simulink model "MGTestSystem_4bus"  (R2021b)
settings: Solver=VariableStepAuto  StartTime=0.0  StopTime=4  RelTol=1e-3
PreLoadFcn:
  | addpath Icons
  | addpath Util
InitFcn:
  | clc
  | %clear all
  | 
  | nDER = 4;
  | xssum = zeros(nDER*2,1);
  | save XSSUM xssum
  | 
  | Ts_Control=1e-4;       % local control time step
  | Ts_Simulation=5e-5;   %simulation time step
  | Ts_Power=5e-5;   % measurement time step
  | Tdisc=0.8;     % time setting for disconnecting from the main grid
  | 
  | Iref = 0.3;  % in p.u.
  | Iqref = 0;  % in p.u.
  | 
  | Ts_secondary =3e-2;   %  secondary control time step
  | %Ts_PMU = 1/60;
  | 
  | ft2km=3.0480e-04;
  | 
  | KPdroop=3.4e-4;
  | KQdroop=1e-3/1;
  | KPdroop2=4.5e-4;
  | KQdroop2=1.5e-3/1;
  | 
  | %KWinvdroop = 20.0;
  | %KVinvdroop = 16.7;
  | %KWinvdroop = 0.05;
  | %KVinvdroop = 0.08;
  | 
  | KWinvdroop = 1/(2*pi*KPdroop);
  | KVinvdroop = 1/(2*pi*KQdroop)
  | KWinvdroop2 = 1/(2*pi*KPdroop2);
  | KVinvdroop2 = 1/(2*pi*KQdroop2)
  | %KVinvdroop = 1/(KQdroop);
  | %KVinvdroop2 = 1/(KQdroop2);
  | %KWinvdroop = 1/(KPdroop);
  | %KWinvdroop2 = 1/(KPdroop2);
  | 
  | droopv1=1/KVinvdroop
  | droopv2=1/KVinvdroop2
  | 
  | 
  | 
  | 
  | wfilter = 35;
  | Rv=0.0;
  | Lv=0e-3;
  | 
  | div=1;
  | 
  | 
  | Kpac=0.1/1;
  | Kiac=420/1;
  | Kpaci=15/div;
  | Kiaci=2e3/div;
  | Kpac2=0.05/1;
  | Kiac2=390/1;
  | Kpaci2=15/div;
  | Kiaci2=1.6e3/div;
  | ... (+47 lines)
undefined symbols (not defined in the file or in its folder): D1, Delta, Ion, Lithium
libraries: spsStairGeneratorLib x24, spsThreePhaseSeriesRLCBranchLib x24, powerlib_extras x23, spsSeriesRLCBranchLib x20, spsThreePhaseVIMeasurementLib x18, slpidlib x18, spsThreePhaseBreakerLib x15, spsRMSLib x10, spsThreePhaseSeriesRLCLoadLib x8, spsVoltageMeasurementLib x8, spsPMUPLLBasedPositiveSequenceLib x6, spsPowerLib x5
(part 2 of 7)

== system MGTestSystem_4bus/DER 1 ==
  Battery : spsBatteryLib/Battery  Commented=on  BatType=Lithium-Ion  ShowTempParam=off  ThermalPreset=no  ShowAgeParam=off  NomV=960  NomQ=10  SOC=75  Batt_Tr=30  PresetModel=on  MaxQ=10  MinV=720  FullV=1117.4277  Dis_rate=4.3478  R=0.96  Normal_OP=9.0435  expZone="[1037.1704     0.49130435]"  current=[6.5 13 32.5]  Units=Time  Tci=20  NomT=20  T2=-30  MaxQ2=4.8  FullV2=7.1  Normal_OP2=5.655  expZone2="[6.58           1]"  Rca=0.6  ti=2000  Dp=0  Neq0=0  Tsim=1e6  Ta1=25  Qeol=5.4*0.9  Reol=0.013333*1.2  Char_age=[2.3478, 3]  Dis_age=[2.3478, 10]  N1=1500  N2=10500  N3=1000  N4=1400  Ta2=45  N5=950
  C1 : spsSeriesRLCBranchLib/Series RLC Branch  LConnTagsString=__new0  RConnTagsString=__new0  BranchType=C  Resistance=1.0  Inductance=1.0  SetiL0=off  InitialCurrent=0  Capacitance=50e-3  Setx0=off  InitialVoltage=960  Measurements=None
  C2 : spsSeriesRLCBranchLib/Series RLC Branch  LConnTagsString=__new0  RConnTagsString=__new0  BranchType=R  Resistance=1e-9  Inductance=1.0  SetiL0=off  InitialCurrent=0  Capacitance=200e-3  Setx0=on  InitialVoltage=500  Measurements=None
  DC Voltage Source : spsDCVoltageSourceLib/DC Voltage Source  Amplitude=VDC  Measurements=None
  DC/DC 1 : Subsystem  Commented=on
  Demux : Demux  Commented=on  Outputs=3
  Irradiance (W/m2) 1 : spsStairGeneratorLib/Stair Generator  Commented=on  t=[0, 10.5, 12.3]  e=[1,0.05, 1.0]*1000  Ts=Ts_Power
  L : spsThreePhaseSeriesRLCBranchLib/Three-Phase Series RLC Branch  LConnTagsString=A|B|C  RConnTagsString=A|B|C  BranchType=RL  Resistance=0.1  Inductance=1.35e-3  Capacitance=inf  Measurements=None
  L1 : spsThreePhaseSeriesRLCBranchLib/Three-Phase Series RLC Branch  LConnTagsString=A|B|C  RConnTagsString=A|B|C  BranchType=RC  Resistance=1  Inductance=3.9e-3  Capacitance=50e-6  Measurements=None
  L3 : spsThreePhaseSeriesRLCBranchLib/Three-Phase Series RLC Branch  Commented=on  LConnTagsString=A|B|C  RConnTagsString=A|B|C  BranchType=RL  Resistance=0*0.03  Inductance=0*0.35e-3  Capacitance=1e-9  Measurements=None
  Local bus : spsThreePhaseVIMeasurementLib/Three-Phase V-I Measurement  VoltageMeasurement=phase-to-ground  SetLabelV=off  LabelV=Vgrid  Vpu=off  VpuLL=off  CurrentMeasurement=yes  SetLabelI=off  LabelI=Igrid  Ipu=off  Pbase=100e6  Vbase=500e3  OutputType=Magnitude  PhasorSimulation=off  PSBequivalent=0
  PV Array 1 : spsPVArrayLib/PV Array  Commented=on  Npar=32  Nser=3  PlotType=array @ 1000 W/m2 & specified temperatures  S_vec="[ 1000  500  100 ]"  Temp_C_vec="[ 45 25  ]"  ModuleName=SunPower SPR-315E-WHT-D  PlotWhenSelected=off  Pm=315.072  Ncell=96  Voc=64.6  Isc=6.14  Vm=54.7  Im=5.76  beta_Voc_pc=-0.2727  alpha_Isc_pc=0.061743  beta_Voc=-0.17616  alpha_Isc=0.003791  IL=6.1461  I0=6.5067e-12  nI=0.95071  Rsh=430.0666  Rs=0.43041  RobustModel=off  RobustCellTemperature=313.3991  BAL=off  Tc=1e-6  Tfilter=5e-5
  Rate Limiter2 : RateLimiter  Commented=on  RisingSlewLimit=8000  FallingSlewLimit=-8000  SampleTimeMode=inherited  InitialCondition=1000
  Scope : Scope
  Scope1 : Scope
  Scope2 : Scope  Commented=on  NumInputPorts=3
  VSC (Average Model) : spsUniversalBridgeLib/Universal Bridge  Arms=3  SnubberResistance=1e5  SnubberCapacitance=inf  Device=Average-model based VSC  Ron=1e-3  Lon=0  ForwardVoltages="[  0  0  ]"  ForwardVoltage=0  GTOparameters=[ 10e-6 , 20e-6 ]  IGBTparameters=[ 1e-6 , 2e-6 ]  Measurements=None  Measurements_2=None  converterType=Rectifier
  VSC Control : Subsystem  mask(VSC Main Controller){nom=[ Pvscr 60 ], Vnom=[480 480], Vnom_dc=VDC, RLxfo=[0*0.03*Pvscr/(480^2)  0*0.35e-3*Pvscr/(480^2)*2*pi*60], RLchoke=[0.08  1.35e-3 ], K_VDCreg=[7  800], K_Ireg=[Kpaci Kiaci], Ts=Ts_Control}
      mask prompts: nom "Nominal power and frequency [ Pnom(VA)  Fnom(Hz) ]:"; Vnom "Nominal primary and secondary voltages (Vrms LL) [ Vnom_prim   Vnom_sec ]:"; Vnom_dc "Nominal DC bus voltage (V):"; RLxfo "Total transformer leakage impedance (pu/Pnom) [ Rxfo  Lxf ]"; RLchoke "Choke impedance [ R(ohm) L(H) ]"; K_VDCreg "VDC regultator gains [ Kp  Ki ]:"; K_Ireg "Current regulator gains [ Kp  Ki ]:"; Ts "Sample time"
      mask init:
      | Pnom=nom(1);
      | Fnom=nom(2);
      | Vnom_prim=Vnom(1);
      | Vnom_sec=Vnom(2);
      | Zbase=Vnom_sec^2/Pnom;
      | Rtot_pu=RLxfo(1) + RLchoke(1)/Zbase;
      | Ltot_pu=RLxfo(2) + RLchoke(2)/(Zbase/(2*pi*Fnom));
      | Kp_VDCreg=K_VDCreg(1);
      | Ki_VDCreg=K_VDCreg(2);
      | Kp_Ireg=K_Ireg(1);
      | Ki_Ireg=K_Ireg(2);
      | Vdc_ref=Vnom_dc;
  "Vdc " : spsVoltageMeasurementLib/Voltage Measurement  Tag=PoWeRsYsTeMmEaSuReMeNt  PhasorSimulation=off  OutputType=Magnitude  PSBequivalent=0
  Conn1 : PMIOPort  Side=Left
  Conn2 : PMIOPort  Port=2  Side=Left
  Conn3 : PMIOPort  Port=3  Side=Left
  wires:
  "Vdc "/1 -> Scope/1, VSC Control/3(Vdc)
  VSC Control/1(Uref) -> Scope1/1, VSC (Average Model)/1
  Local bus/1 -> VSC Control/1(V)
  Local bus/2 -> VSC Control/2(I)
  Irradiance (W/m2) 1/1 -> Rate Limiter2/1
  Rate Limiter2/1 -> PV Array 1/1
  PV Array 1/1 -> DC/DC 1/1(m_PV)
  Demux/1 -> Scope2/1
  Demux/3 -> Scope2/3
  Battery/1 -> Demux/1
  Demux/2 -> Scope2/2
  connections:
  VSC (Average Model)/LConn2 -- L/LConn2
  VSC (Average Model)/LConn3 -- L/LConn3
  VSC (Average Model)/LConn1 -- L/LConn1
  "Vdc "/LConn1 -- C2/LConn1 -- C1/LConn1 -- VSC (Average Model)/RConn1
  VSC (Average Model)/RConn2 -- "Vdc "/LConn2 -- C1/RConn1 -- DC/DC 1/RConn2 -- Battery/LConn2 -- DC Voltage Source/LConn1
  Local bus/LConn3 -- L1/LConn3 -- L/RConn3
  Local bus/RConn1 -- Conn1/RConn1
  Local bus/RConn2 -- Conn2/RConn1
  Local bus/RConn3 -- Conn3/RConn1
  DC Voltage Source/RConn1 -- Battery/LConn1 -- DC/DC 1/RConn1 -- C2/RConn1
  PV Array 1/RConn2 -- DC/DC 1/LConn2
  PV Array 1/RConn1 -- DC/DC 1/LConn1
  L/RConn1 -- Local bus/LConn1 -- L1/LConn1
  L/RConn2 -- Local bus/LConn2 -- L1/LConn2
  L1/RConn2 -- L1/RConn3 -- L1/RConn1

== system MGTestSystem_4bus/DER 2 ==
  C1 : spsSeriesRLCBranchLib/Series RLC Branch  LConnTagsString=__new0  RConnTagsString=__new0  BranchType=C  Resistance=1.0  Inductance=1.0  SetiL0=off  InitialCurrent=0  Capacitance=200e-3  Setx0=off  InitialVoltage=900  Measurements=None
  C2 : spsSeriesRLCBranchLib/Series RLC Branch  LConnTagsString=__new0  RConnTagsString=__new0  BranchType=R  Resistance=1e-9  Inductance=1.0  SetiL0=off  InitialCurrent=0  Capacitance=200e-3  Setx0=on  InitialVoltage=500  Measurements=None
  DC Voltage Source : spsDCVoltageSourceLib/DC Voltage Source  Amplitude=VDC  Measurements=None
  DC/DC 1 : Subsystem  Commented=on
  Irradiance (W/m2) 1 : spsStairGeneratorLib/Stair Generator  Commented=on  t=[0, 10.5, 12.3]  e=[1,0.05, 1.0]*1000  Ts=Ts_Power
  L : spsThreePhaseSeriesRLCBranchLib/Three-Phase Series RLC Branch  LConnTagsString=A|B|C  RConnTagsString=A|B|C  BranchType=RL  Resistance=0.1  Inductance=1.35e-3  Capacitance=inf  Measurements=None
  L1 : spsThreePhaseSeriesRLCBranchLib/Three-Phase Series RLC Branch  LConnTagsString=A|B|C  RConnTagsString=A|B|C  BranchType=RC  Resistance=1  Inductance=3.9e-3  Capacitance=50e-6  Measurements=None
  L3 : spsThreePhaseSeriesRLCBranchLib/Three-Phase Series RLC Branch  Commented=on  LConnTagsString=A|B|C  RConnTagsString=A|B|C  BranchType=RL  Resistance=0*0.03  Inductance=0*0.35e-3  Capacitance=1e-9  Measurements=None
  PV Array 1 : spsPVArrayLib/PV Array  Commented=on  Npar=32  Nser=3  PlotType=array @ 1000 W/m2 & specified temperatures  S_vec="[ 1000  500  100 ]"  Temp_C_vec="[ 45 25  ]"  ModuleName=SunPower SPR-315E-WHT-D  PlotWhenSelected=off  Pm=315.072  Ncell=96  Voc=64.6  Isc=6.14  Vm=54.7  Im=5.76  beta_Voc_pc=-0.2727  alpha_Isc_pc=0.061743  beta_Voc=-0.17616  alpha_Isc=0.003791  IL=6.1461  I0=6.5067e-12  nI=0.95071  Rsh=430.0666  Rs=0.43041  RobustModel=off  RobustCellTemperature=313.3991  BAL=off  Tc=1e-6  Tfilter=5e-5
  Rate Limiter2 : RateLimiter  Commented=on  RisingSlewLimit=8000  FallingSlewLimit=-8000  SampleTimeMode=inherited  InitialCondition=1000
  Scope : Scope
  VSC (Average Model) : spsUniversalBridgeLib/Universal Bridge  Arms=3  SnubberResistance=1e5  SnubberCapacitance=inf  Device=Average-model based VSC  Ron=1e-3  Lon=0  ForwardVoltages="[  0  0  ]"  ForwardVoltage=0  GTOparameters=[ 10e-6 , 20e-6 ]  IGBTparameters=[ 1e-6 , 2e-6 ]  Measurements=None  Measurements_2=None  converterType=Rectifier
  VSC Control : Subsystem  mask(VSC Main Controller){nom=[ Pvscr 60 ], Vnom=[ 480 480 ], Vnom_dc=VDC, RLxfo=[0*0.03*Pvscr/(480^2)  0*0.35e-3*Pvscr/(480^2)*2*pi*60], RLchoke=[0.1  1.35e-3 ], K_VDCreg=[7  800], K_Ireg=[Kpaci Kiaci], Ts=Ts_Control}
      mask prompts: nom "Nominal power and frequency [ Pnom(VA)  Fnom(Hz) ]:"; Vnom "Nominal primary and secondary voltages (Vrms LL) [ Vnom_prim   Vnom_sec ]:"; Vnom_dc "Nominal DC bus voltage (V):"; RLxfo "Total transformer leakage impedance (pu/Pnom) [ Rxfo  Lxf ]"; RLchoke "Choke impedance [ R(ohm) L(H) ]"; K_VDCreg "VDC regultator gains [ Kp  Ki ]:"; K_Ireg "Current regulator gains [ Kp  Ki ]:"; Ts "Sample time"
      mask init: same as MGTestSystem_4bus/DER 1/VSC Control
  "Vdc " : spsVoltageMeasurementLib/Voltage Measurement  Tag=PoWeRsYsTeMmEaSuReMeNt  PhasorSimulation=off  OutputType=Magnitude  PSBequivalent=0
  local bus : spsThreePhaseVIMeasurementLib/Three-Phase V-I Measurement  VoltageMeasurement=phase-to-ground  SetLabelV=off  LabelV=Vgrid  Vpu=off  VpuLL=off  CurrentMeasurement=yes  SetLabelI=off  LabelI=Igrid  Ipu=off  Pbase=100e6  Vbase=500e3  OutputType=Magnitude  PhasorSimulation=off  PSBequivalent=0
  Conn1 : PMIOPort  Side=Left
  Conn2 : PMIOPort  Port=2  Side=Left
  Conn3 : PMIOPort  Port=3  Side=Left
  wires:
  "Vdc "/1 -> Scope/1, VSC Control/3(Vdc)
  VSC Control/1(Uref) -> VSC (Average Model)/1
  local bus/1 -> VSC Control/1(V)
  local bus/2 -> VSC Control/2(I)
  Irradiance (W/m2) 1/1 -> Rate Limiter2/1
  Rate Limiter2/1 -> PV Array 1/1
  PV Array 1/1 -> DC/DC 1/1(m_PV)
  connections:
  VSC (Average Model)/LConn2 -- L/LConn2
  VSC (Average Model)/LConn3 -- L/LConn3
  VSC (Average Model)/LConn1 -- L/LConn1
  L/RConn2 -- L1/LConn2 -- local bus/LConn2
  "Vdc "/LConn1 -- C2/LConn1 -- C1/LConn1 -- VSC (Average Model)/RConn1
  VSC (Average Model)/RConn2 -- "Vdc "/LConn2 -- C1/RConn1 -- DC/DC 1/RConn2 -- DC Voltage Source/LConn1
  local bus/RConn1 -- Conn1/RConn1
  local bus/RConn2 -- Conn2/RConn1
  local bus/RConn3 -- Conn3/RConn1
  DC Voltage Source/RConn1 -- DC/DC 1/RConn1 -- C2/RConn1
  L1/RConn3 -- L1/RConn1 -- L1/RConn2
  PV Array 1/RConn2 -- DC/DC 1/LConn2
  PV Array 1/RConn1 -- DC/DC 1/LConn1
  L/RConn1 -- local bus/LConn1 -- L1/LConn1
  L/RConn3 -- L1/LConn3 -- local bus/LConn3

== system MGTestSystem_4bus/DER 3 ==
  C1 : spsSeriesRLCBranchLib/Series RLC Branch  LConnTagsString=__new0  RConnTagsString=__new0  BranchType=C  Resistance=1.0  Inductance=1.0  SetiL0=off  InitialCurrent=0  Capacitance=50e-3  Setx0=off  InitialVoltage=960  Measurements=None
  C2 : spsSeriesRLCBranchLib/Series RLC Branch  LConnTagsString=__new0  RConnTagsString=__new0  BranchType=R  Resistance=1e-9  Inductance=1.0  SetiL0=off  InitialCurrent=0  Capacitance=200e-3  Setx0=on  InitialVoltage=500  Measurements=None
  DC Voltage Source : spsDCVoltageSourceLib/DC Voltage Source  Amplitude=VDC  Measurements=None
  DC/DC 1 : Subsystem  Commented=on
  Irradiance (W/m2) 1 : spsStairGeneratorLib/Stair Generator  Commented=on  t=[0, 10.5, 12.3]  e=[1,0.05, 1.0]*1000  Ts=Ts_Power
  L : spsThreePhaseSeriesRLCBranchLib/Three-Phase Series RLC Branch  LConnTagsString=A|B|C  RConnTagsString=A|B|C  BranchType=RL  Resistance=0.1  Inductance=1.35e-3  Capacitance=inf  Measurements=None
  L1 : spsThreePhaseSeriesRLCBranchLib/Three-Phase Series RLC Branch  LConnTagsString=A|B|C  RConnTagsString=A|B|C  BranchType=RC  Resistance=1  Inductance=3.9e-3  Capacitance=50e-6  Measurements=None
  L3 : spsThreePhaseSeriesRLCBranchLib/Three-Phase Series RLC Branch  Commented=on  LConnTagsString=A|B|C  RConnTagsString=A|B|C  BranchType=RL  Resistance=0*0.04  Inductance=0*0.46e-3  Capacitance=1e-9  Measurements=None
  PV Array 1 : spsPVArrayLib/PV Array  Commented=on  Npar=32  Nser=3  PlotType=array @ 1000 W/m2 & specified temperatures  S_vec="[ 1000  500  100 ]"  Temp_C_vec="[ 45 25  ]"  ModuleName=SunPower SPR-315E-WHT-D  PlotWhenSelected=off  Pm=315.072  Ncell=96  Voc=64.6  Isc=6.14  Vm=54.7  Im=5.76  beta_Voc_pc=-0.2727  alpha_Isc_pc=0.061743  beta_Voc=-0.17616  alpha_Isc=0.003791  IL=6.1461  I0=6.5067e-12  nI=0.95071  Rsh=430.0666  Rs=0.43041  RobustModel=off  RobustCellTemperature=313.3991  BAL=off  Tc=1e-6  Tfilter=5e-5
  Rate Limiter2 : RateLimiter  Commented=on  RisingSlewLimit=8000  FallingSlewLimit=-8000  SampleTimeMode=inherited  InitialCondition=1000
  Scope : Scope
  VSC (Average Model) : spsUniversalBridgeLib/Universal Bridge  Arms=3  SnubberResistance=1e5  SnubberCapacitance=inf  Device=Average-model based VSC  Ron=1e-3  Lon=0  ForwardVoltages="[  0  0  ]"  ForwardVoltage=0  GTOparameters=[ 10e-6 , 20e-6 ]  IGBTparameters=[ 1e-6 , 2e-6 ]  Measurements=None  Measurements_2=None  converterType=Rectifier
  VSC Control : Subsystem  mask(VSC Main Controller){nom=[ Pvscr 60 ], Vnom=[ 480 480 ], Vnom_dc=VDC, RLxfo=[0*0.04*Pvscr/(480^2)  0*0.46e-3*Pvscr/(480^2)*2*pi*60], RLchoke=[0.1  1.35e-3], K_VDCreg=[7  800], K_Ireg=[Kpaci2 Kiaci2], Ts=Ts_Control}
      mask prompts: nom "Nominal power and frequency [ Pnom(VA)  Fnom(Hz) ]:"; Vnom "Nominal primary and secondary voltages (Vrms LL) [ Vnom_prim   Vnom_sec ]:"; Vnom_dc "Nominal DC bus voltage (V):"; RLxfo "Total transformer leakage impedance (pu/Pnom) [ Rxfo  Lxf ]"; RLchoke "Choke impedance [ R(ohm) L(H) ]"; K_VDCreg "VDC regultator gains [ Kp  Ki ]:"; K_Ireg "Current regulator gains [ Kp  Ki ]:"; Ts "Sample time"
      mask init: same as MGTestSystem_4bus/DER 1/VSC Control
  "Vdc " : spsVoltageMeasurementLib/Voltage Measurement  Tag=PoWeRsYsTeMmEaSuReMeNt  PhasorSimulation=off  OutputType=Magnitude  PSBequivalent=0
  grid : spsThreePhaseVIMeasurementLib/Three-Phase V-I Measurement  VoltageMeasurement=phase-to-ground  SetLabelV=off  LabelV=Vgrid  Vpu=off  VpuLL=off  CurrentMeasurement=yes  SetLabelI=off  LabelI=Igrid  Ipu=off  Pbase=100e6  Vbase=500e3  OutputType=Magnitude  PhasorSimulation=off  PSBequivalent=0
  Conn1 : PMIOPort  Side=Left
  Conn2 : PMIOPort  Port=2  Side=Left
  Conn3 : PMIOPort  Port=3  Side=Left
  wires:
  "Vdc "/1 -> Scope/1, VSC Control/3(Vdc)
  VSC Control/1(Uref) -> VSC (Average Model)/1
  grid/1 -> VSC Control/1(V)
  grid/2 -> VSC Control/2(I)
  Irradiance (W/m2) 1/1 -> Rate Limiter2/1
  Rate Limiter2/1 -> PV Array 1/1
  PV Array 1/1 -> DC/DC 1/1(m_PV)
  connections:
  VSC (Average Model)/LConn2 -- L/LConn2
  VSC (Average Model)/LConn3 -- L/LConn3
  VSC (Average Model)/LConn1 -- L/LConn1
  L/RConn3 -- L1/LConn3 -- grid/LConn3
  L/RConn2 -- L1/LConn2 -- grid/LConn2
  "Vdc "/LConn1 -- C2/LConn1 -- C1/LConn1 -- VSC (Average Model)/RConn1
  VSC (Average Model)/RConn2 -- "Vdc "/LConn2 -- C1/RConn1 -- DC Voltage Source/LConn1 -- DC/DC 1/RConn2
  grid/RConn1 -- Conn1/RConn1
  grid/RConn2 -- Conn2/RConn1
  grid/RConn3 -- Conn3/RConn1
  DC Voltage Source/RConn1 -- DC/DC 1/RConn1 -- C2/RConn1
  L1/RConn3 -- L1/RConn1 -- L1/RConn2
  PV Array 1/RConn2 -- DC/DC 1/LConn2
  PV Array 1/RConn1 -- DC/DC 1/LConn1
  L/RConn1 -- grid/LConn1 -- L1/LConn1

== system MGTestSystem_4bus/DER 4 ==
  Battery : spsBatteryLib/Battery  Commented=on  BatType=Lithium-Ion  ShowTempParam=off  ThermalPreset=no  ShowAgeParam=off  NomV=850  NomQ=100  SOC=50  Batt_Tr=30  PresetModel=on  MaxQ=100  MinV=637.5  FullV=989.3891  Dis_rate=43.4783  R=0.085  Normal_OP=90.4348  expZone="[918.328      4.913043]"  current=[6.5 13 32.5]  Units=Time  Tci=20  NomT=20  T2=-30  MaxQ2=4.8  FullV2=7.1  Normal_OP2=5.655  expZone2="[6.58           1]"  Rca=0.6  ti=2000  Dp=0  Neq0=0  Tsim=1e6  Ta1=25  Qeol=5.4*0.9  Reol=0.013333*1.2  Char_age=[2.3478, 3]  Dis_age=[2.3478, 10]  N1=1500  N2=10500  N3=1000  N4=1400  Ta2=45  N5=950
  C1 : spsSeriesRLCBranchLib/Series RLC Branch  LConnTagsString=__new0  RConnTagsString=__new0  BranchType=C  Resistance=1.0  Inductance=1.0  SetiL0=off  InitialCurrent=0  Capacitance=200e-3  Setx0=off  InitialVoltage=900  Measurements=None
  C2 : spsSeriesRLCBranchLib/Series RLC Branch  LConnTagsString=__new0  RConnTagsString=__new0  BranchType=R  Resistance=1e-9  Inductance=1.0  SetiL0=off  InitialCurrent=0  Capacitance=200e-3  Setx0=on  InitialVoltage=500  Measurements=None
  DC Voltage Source : spsDCVoltageSourceLib/DC Voltage Source  Amplitude=VDC  Measurements=None
  DC/DC 1 : Subsystem  Commented=on
  Demux : Demux  Commented=on  Outputs=3
  Irradiance (W/m2) 1 : spsStairGeneratorLib/Stair Generator  Commented=on  t=[0, 10.5, 12.3]  e=[1,0.05, 1.0]*1000  Ts=Ts_Power
  L : spsThreePhaseSeriesRLCBranchLib/Three-Phase Series RLC Branch  LConnTagsString=A|B|C  RConnTagsString=A|B|C  BranchType=RL  Resistance=0.1  Inductance=1.35e-3  Capacitance=inf  Measurements=None
  L1 : spsThreePhaseSeriesRLCBranchLib/Three-Phase Series RLC Branch  LConnTagsString=A|B|C  RConnTagsString=A|B|C  BranchType=RC  Resistance=1  Inductance=3.9e-3  Capacitance=50e-6  Measurements=None
  L3 : spsThreePhaseSeriesRLCBranchLib/Three-Phase Series RLC Branch  Commented=on  LConnTagsString=A|B|C  RConnTagsString=A|B|C  BranchType=RL  Resistance=0*0.04  Inductance=0*0.46e-3  Capacitance=1e-9  Measurements=None
  PV Array 1 : spsPVArrayLib/PV Array  Commented=on  Npar=32  Nser=3  PlotType=array @ 1000 W/m2 & specified temperatures  S_vec="[ 1000  500  100 ]"  Temp_C_vec="[ 45 25  ]"  ModuleName=SunPower SPR-315E-WHT-D  PlotWhenSelected=off  Pm=315.072  Ncell=96  Voc=64.6  Isc=6.14  Vm=54.7  Im=5.76  beta_Voc_pc=-0.2727  alpha_Isc_pc=0.061743  beta_Voc=-0.17616  alpha_Isc=0.003791  IL=6.1461  I0=6.5067e-12  nI=0.95071  Rsh=430.0666  Rs=0.43041  RobustModel=off  RobustCellTemperature=313.3991  BAL=off  Tc=1e-6  Tfilter=5e-5
  Rate Limiter2 : RateLimiter  Commented=on  RisingSlewLimit=8000  FallingSlewLimit=-8000  SampleTimeMode=inherited  InitialCondition=1000
  Scope : Scope
  Scope1 : Scope  Commented=on  NumInputPorts=3
  VSC (Average Model) : spsUniversalBridgeLib/Universal Bridge  Arms=3  SnubberResistance=1e5  SnubberCapacitance=inf  Device=Average-model based VSC  Ron=1e-3  Lon=0  ForwardVoltages="[  0  0  ]"  ForwardVoltage=0  GTOparameters=[ 10e-6 , 20e-6 ]  IGBTparameters=[ 1e-6 , 2e-6 ]  Measurements=None  Measurements_2=None  converterType=Rectifier
  VSC Control : Subsystem  mask(VSC Main Controller){nom=[ Pvscr 60 ], Vnom=[ 480 480 ], Vnom_dc=VDC, RLxfo=[0*0.04*Pvscr/(480^2)  0*0.46e-3*Pvscr/(480^2)*2*pi*60], RLchoke=[0.1  1.35e-3], K_VDCreg=[7  800], K_Ireg=[Kpaci2 Kiaci2], Ts=Ts_Control}
      mask prompts: nom "Nominal power and frequency [ Pnom(VA)  Fnom(Hz) ]:"; Vnom "Nominal primary and secondary voltages (Vrms LL) [ Vnom_prim   Vnom_sec ]:"; Vnom_dc "Nominal DC bus voltage (V):"; RLxfo "Total transformer leakage impedance (pu/Pnom) [ Rxfo  Lxf ]"; RLchoke "Choke impedance [ R(ohm) L(H) ]"; K_VDCreg "VDC regultator gains [ Kp  Ki ]:"; K_Ireg "Current regulator gains [ Kp  Ki ]:"; Ts "Sample time"
      mask init: same as MGTestSystem_4bus/DER 1/VSC Control
  "Vdc " : spsVoltageMeasurementLib/Voltage Measurement  Tag=PoWeRsYsTeMmEaSuReMeNt  PhasorSimulation=off  OutputType=Magnitude  PSBequivalent=0
  grid : spsThreePhaseVIMeasurementLib/Three-Phase V-I Measurement  VoltageMeasurement=phase-to-ground  SetLabelV=off  LabelV=Vgrid  Vpu=off  VpuLL=off  CurrentMeasurement=yes  SetLabelI=off  LabelI=Igrid  Ipu=off  Pbase=100e6  Vbase=500e3  OutputType=Magnitude  PhasorSimulation=off  PSBequivalent=0
  Conn1 : PMIOPort  Side=Left
  Conn2 : PMIOPort  Port=2  Side=Left
  Conn3 : PMIOPort  Port=3  Side=Left
  wires:
  grid/2 -> VSC Control/2(I)
  grid/1 -> VSC Control/1(V)
  VSC Control/1(Uref) -> VSC (Average Model)/1
  "Vdc "/1 -> VSC Control/3(Vdc), Scope/1
  Demux/1 -> Scope1/1
  Battery/1 -> Demux/1
  Demux/3 -> Scope1/3
  Demux/2 -> Scope1/2
  Irradiance (W/m2) 1/1 -> Rate Limiter2/1
  PV Array 1/1 -> DC/DC 1/1(m_PV)
  Rate Limiter2/1 -> PV Array 1/1
  connections:
  L1/RConn2 -- L1/RConn1 -- L1/RConn3
  DC Voltage Source/RConn1 -- DC/DC 1/RConn1 -- Battery/LConn1 -- C2/RConn1
  grid/RConn3 -- Conn3/RConn1
  grid/RConn2 -- Conn2/RConn1
  grid/RConn1 -- Conn1/RConn1
  L/RConn3 -- L1/LConn3 -- grid/LConn3
  C1/RConn1 -- "Vdc "/LConn2 -- VSC (Average Model)/RConn2 -- DC/DC 1/RConn2 -- Battery/LConn2 -- DC Voltage Source/LConn1
  VSC (Average Model)/RConn1 -- C1/LConn1 -- C2/LConn1 -- "Vdc "/LConn1
  L/RConn2 -- grid/LConn2 -- L1/LConn2
  VSC (Average Model)/LConn1 -- L/LConn1
  VSC (Average Model)/LConn3 -- L/LConn3
  VSC (Average Model)/LConn2 -- L/LConn2
  L/RConn1 -- grid/LConn1 -- L1/LConn1
  PV Array 1/RConn2 -- DC/DC 1/LConn2
  PV Array 1/RConn1 -- DC/DC 1/LConn1

== system MGTestSystem_4bus/Grid-Connected Battery (EMT with Simple Controls) ==
  PQref : Inport  SampleTime=Ts_Control
  Battery : spsBatteryLib/Battery  BatType=Lithium-Ion  ShowTempParam=off  ThermalPreset=no  ShowAgeParam=off  NomV=Vnom_dc  NomQ=Bcap  SOC=75  Batt_Tr=30  PresetModel=on  MaxQ=100  MinV=360  FullV=558.7138  Dis_rate=43.4783  R=0.048  Normal_OP=90.4348  expZone="[518.5852      4.913043]"  current=[6.5 13 32.5]  Units=Time  Tci=20  NomT=25  T2=0  MaxQ2=2.208  FullV2=3.45  Normal_OP2=2.8  expZone2="[3.22        0.23]"  Rca=0.6  ti=1000  Dp=0  Neq0=0  Tsim=1e6  Ta1=25  Qeol=5.4*0.9  Reol=0.013333*1.2  Char_age=[2.3478, 3]  Dis_age=[2.3478, 10]  N1=1500  N2=10500  N3=1000  N4=1400  Ta2=45  N5=950
  Battery Controller : Subsystem  SystemSampleTime=Ts
  Bus Selector : BusSelector  OutputSignals=Vabc,Iabc
  DC Link : Subsystem
  Grid Inverter : Subsystem
  Inverter Control : Subsystem
  Measures : Subsystem
  Rate Transition2 : RateTransition  OutPortSampleTime=Ts_Control
  A : PMIOPort  Side=Right
  B : PMIOPort  Port=2  Side=Right
  C : PMIOPort  Port=3  Side=Right
  m : Outport  VectorParamsAs1DForOutWhenUnconnected=off
  wires:
  Battery Controller/1(Idq_ref) -> Inverter Control/3(Idq_ref)
  [m_inv] -> Rate Transition2/1
  Battery/1 -> [m_batt]
  Measures/1(m) -> m/1
  [m_batt] -> Measures/2(Battery)
  [m_inv] -> Measures/1(Grid)
  Grid Inverter/1(m) -> [m_inv]
  Bus Selector/2 -> Inverter Control/2(Iabc_prim)  "<Iabc>"
  Bus Selector/1 -> Inverter Control/1(Vabc_prim)  "<Vabc>"
  Inverter Control/1(Uref) -> Grid Inverter/1(Uref)
  Rate Transition2/1 -> Bus Selector/1, Battery Controller/1(m)
  PQref/1 -> Battery Controller/2(PQref)
  connections:
  DC Link/RConn2 -- Grid Inverter/LConn2
  Grid Inverter/LConn1 -- DC Link/RConn1
  C/RConn1 -- Grid Inverter/RConn3
  B/RConn1 -- Grid Inverter/RConn2
  A/RConn1 -- Grid Inverter/RConn1
  Grid Inverter/LConn3 -- DC Link/RConn3
  Battery/LConn2 -- DC Link/LConn2
  Battery/LConn1 -- DC Link/LConn1

== system MGTestSystem_4bus/Grid-Connected Battery (EMT with Simple Controls)1 ==
  PQref : Inport  SampleTime=Ts_Control
  Battery : spsBatteryLib/Battery  BatType=Lithium-Ion  ShowTempParam=off  ThermalPreset=no  ShowAgeParam=off  NomV=Vnom_dc  NomQ=Bcap  SOC=75  Batt_Tr=30  PresetModel=on  MaxQ=100  MinV=360  FullV=558.7138  Dis_rate=43.4783  R=0.048  Normal_OP=90.4348  expZone="[518.5852      4.913043]"  current=[6.5 13 32.5]  Units=Time  Tci=20  NomT=25  T2=0  MaxQ2=2.208  FullV2=3.45  Normal_OP2=2.8  expZone2="[3.22        0.23]"  Rca=0.6  ti=1000  Dp=0  Neq0=0  Tsim=1e6  Ta1=25  Qeol=5.4*0.9  Reol=0.013333*1.2  Char_age=[2.3478, 3]  Dis_age=[2.3478, 10]  N1=1500  N2=10500  N3=1000  N4=1400  Ta2=45  N5=950
  Battery Controller : Subsystem  SystemSampleTime=Ts
  Bus Selector : BusSelector  OutputSignals=Vabc,Iabc
  DC Link : Subsystem
  Grid Inverter : Subsystem
  Inverter Control : Subsystem
  Measures : Subsystem
  Rate Transition2 : RateTransition  OutPortSampleTime=Ts_Control
  A : PMIOPort  Side=Right
  B : PMIOPort  Port=2  Side=Right
  C : PMIOPort  Port=3  Side=Right
  m : Outport  VectorParamsAs1DForOutWhenUnconnected=off
  wires:
  Battery Controller/1(Idq_ref) -> Inverter Control/3(Idq_ref)
  [m_inv] -> Rate Transition2/1
  Battery/1 -> [m_batt]
  Measures/1(m) -> m/1
  [m_batt] -> Measures/2(Battery)
  [m_inv] -> Measures/1(Grid)
  Grid Inverter/1(m) -> [m_inv]
  Bus Selector/2 -> Inverter Control/2(Iabc_prim)  "<Iabc>"
  Bus Selector/1 -> Inverter Control/1(Vabc_prim)  "<Vabc>"
  Inverter Control/1(Uref) -> Grid Inverter/1(Uref)
  Rate Transition2/1 -> Bus Selector/1, Battery Controller/1(m)
  PQref/1 -> Battery Controller/2(PQref)
  connections:
  DC Link/RConn2 -- Grid Inverter/LConn2
  Grid Inverter/LConn1 -- DC Link/RConn1
  C/RConn1 -- Grid Inverter/RConn3
  B/RConn1 -- Grid Inverter/RConn2
  A/RConn1 -- Grid Inverter/RConn1
  Grid Inverter/LConn3 -- DC Link/RConn3
  Battery/LConn2 -- DC Link/LConn2
  Battery/LConn1 -- DC Link/LConn1

== system MGTestSystem_4bus/Main Grid  ==
  note: Thevenin equivalent
  4.16kV : spsThreePhaseSeriesRLCBranchLib/Three-Phase Series RLC Branch  LConnTagsString=A|B|C  RConnTagsString=A|B|C  BranchType=RL  Resistance=4.16e3^2/20e6/10  Inductance=4.16e3^2/20e6/(2*pi*60)  Capacitance=1.0  Measurements=None
  Ground1 : spsGroundLib/Ground  LConnTagsString=a
  Programmable Voltage Source : spsThreePhaseProgrammableVoltageSourceLib/Three-Phase Programmable Voltage Source  PositiveSequence="[4.16e3 0  60]"  VariationEntity=None  VariationType=Table of time-amplitude pairs  VariationTypeAlt=Step  VariationStep=-0.3  VariationRate=0.5  VariationMagnitude=0.4  VariationFrequency=2  VariationTiming=[0.1 1.2]  VariationPhaseA=off  Amplitudes=[1]  TimeValues=[0]  HarmonicGeneration=off  HarmonicA=[3 0.2 -25 0]  HarmonicB="[2 0.15  35 2]"  Timing="[0.1  0.6]"  BusType=swing  Pref=0  Qref=0  Qmin=-inf  Qmax=inf
  C : PMIOPort  Side=Right
  B : PMIOPort  Port=2  Side=Right
  A : PMIOPort  Port=3  Side=Right
  connections:
  Programmable Voltage Source/RConn3 -- 4.16kV/LConn3
  Ground1/LConn1 -- Programmable Voltage Source/LConn1
  Programmable Voltage Source/RConn2 -- 4.16kV/LConn2
  4.16kV/LConn1 -- Programmable Voltage Source/RConn1
  4.16kV/RConn3 -- C/RConn1
  4.16kV/RConn2 -- B/RConn1
  4.16kV/RConn1 -- A/RConn1

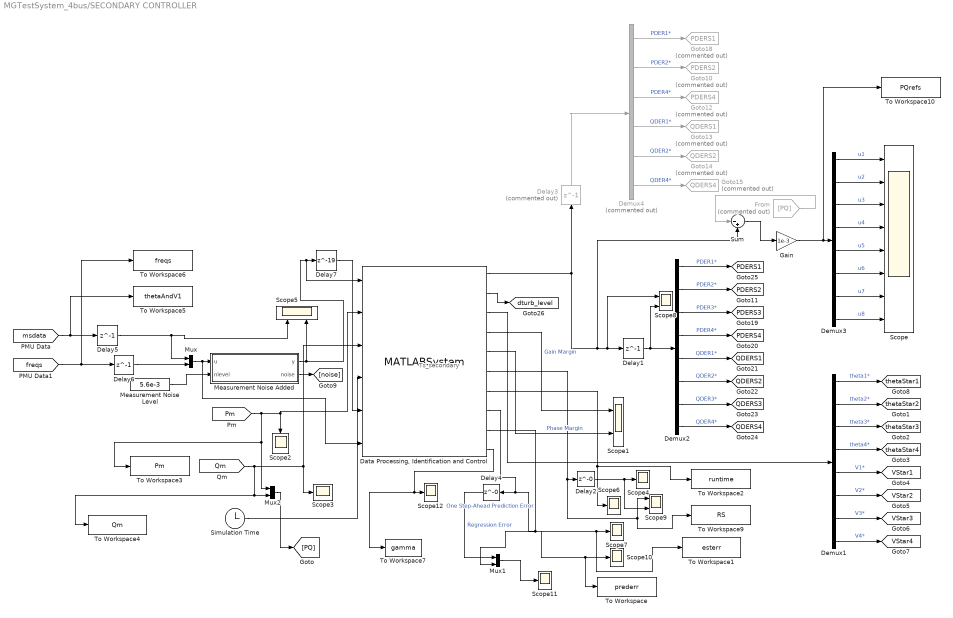
== system MGTestSystem_4bus/SECONDARY CONTROLLER ==
  note: Ts_secondary
  " Measurement Noise Added" : MATLAB Function  TreatAsAtomicUnit=on  SystemSampleTime=Ts_Simulation
  "Data Processing, Identification and Control" : MATLABSystem  System=GlobalIdentControl  Controller=4  Sbase=Pvscr  Vpmax=480/sqrt(3)*sqrt(2)  SampleTime=Ts_secondary*1  ident_window=Ts_secondary*10*1  t_inits=0.0  t_control=Tdisc  kp_droopgain=KPdroop  kq_droopgain=KQdroop  kp_droopgain2=KPdroop2  kq_droopgain2=KQdroop2  PS0=0  QS0=0  ctrlEnabled=1  isOnline=1  qtheta_diag=0  qomega_diag=1e3  qv_diag=1  r=1e-6  smallsignal=0  isNonlinearBases=0  disturbLevel=0.01
      mask Type: GlobalIdentControl
      mask Display:
      | disp('Global Controller');
      | port_label('input',1,'msdata');
      | port_label('input',2,'Pm');
      | port_label('input',3,'Qm');
      | port_label('input',4,'t');
      | port_label('input',5,'msdata_delay');
      | port_label('input',6,'dataactual');
      | port_label('output',1,'P* and Q*');
      | port_label('output',2,'Vref Disturbance');
      | port_label('output',3,'Theta* and V*');
      | port_label('output',4,'Gain Margin');
      | port_label('output',5,'Phase Margin');
      | port_label('output',6,'RS');
      | port_label('output',7,'Run Time (s)');
      | port_label('output',8,'Estimation Error');
      | port_label('output',9,'Prediction Error');
      | port_label('output',10,'gamma');
  Delay1 : Delay  DelayLength=1  InitialCondition=0  SampleTime=0.02*(1+0.1*randn)
  Delay2 : Delay  DelayLength=0  InitialCondition=0  SampleTime=0*Ts_secondary+0.02*(1+0.1*randn)
  Delay3 : Delay  Commented=on  DelayLength=1  InitialCondition=0  SampleTime=0.02*(1+0.1*randn)
  Delay4 : Delay  DelayLength=0  InitialCondition=0  SampleTime=Ts_secondary
  Delay5 : Delay  DelayLength=1  InitialCondition=0  SampleTime=Ts_secondary
  Delay6 : Delay  DelayLength=1  InitialCondition=0  SampleTime=Ts_secondary*1
  Delay7 : Delay  DelayLength=19  InitialCondition=0  SampleTime=Ts_secondary
  Demux1 : Demux  Outputs=8
  Demux2 : Demux  Outputs=8
  Demux3 : Demux  Outputs=8
  Demux4 : Demux  Commented=on  Outputs=6
  From : From  Commented=on  GotoTag=PQ
  Gain : Gain  Gain=1e-3
  Goto10 : Goto  Commented=on  GotoTag=PDERS2  TagVisibility=global
  Goto12 : Goto  Commented=on  GotoTag=PDERS4  TagVisibility=global
  Goto13 : Goto  Commented=on  GotoTag=QDERS1  TagVisibility=global
  Goto14 : Goto  Commented=on  GotoTag=QDERS2  TagVisibility=global
  Goto15 : Goto  Commented=on  GotoTag=QDERS4  TagVisibility=global
  Goto18 : Goto  Commented=on  GotoTag=PDERS1  TagVisibility=global
  Measurement Noise Level : Constant  Value=5.6e-3
  Mux : Mux  Inputs=2
  Mux1 : Mux  Inputs=2
  Mux2 : Mux  Inputs=2
  Scope : Scope  NumInputPorts=8
  Scope{1,5,8..9} (4 alike) : Scope  NumInputPorts=2
  Scope{2..4,6..7,10..12} (8 alike) : Scope
  Simulation Time : Clock
  Sum : Sum  Inputs=|-+
  To Workspace : ToWorkspace  VariableName=prederr  SaveFormat=Structure With Time  SampleTime=-1
      settings: Save2DSignal=2-D array (concatenate along first dimension)
  To Workspace1 : ToWorkspace  VariableName=esterr  SaveFormat=Structure With Time  SampleTime=-1
      settings: Save2DSignal=2-D array (concatenate along first dimension)
  To Workspace10 : ToWorkspace  VariableName=PQrefs  SaveFormat=Structure With Time  SampleTime=-1
      settings: Save2DSignal=2-D array (concatenate along first dimension)
  To Workspace2 : ToWorkspace  VariableName=runtime  SaveFormat=Structure With Time  SampleTime=-1
      settings: Save2DSignal=2-D array (concatenate along first dimension)
  To Workspace3 : ToWorkspace  VariableName=Pm  SaveFormat=Structure With Time  SampleTime=-1
      settings: Save2DSignal=2-D array (concatenate along first dimension)
  To Workspace4 : ToWorkspace  VariableName=Qm  SaveFormat=Structure With Time  SampleTime=-1
      settings: Save2DSignal=2-D array (concatenate along first dimension)
  To Workspace5 : ToWorkspace  VariableName=thetaAndV1  SaveFormat=Structure With Time  SampleTime=-1
      settings: Save2DSignal=2-D array (concatenate along first dimension)
  To Workspace6 : ToWorkspace  VariableName=freqs  SaveFormat=Structure With Time  SampleTime=-1
      settings: Save2DSignal=2-D array (concatenate along first dimension)
  To Workspace7 : ToWorkspace  VariableName=gamma  SaveFormat=Structure With Time  SampleTime=-1
      settings: Save2DSignal=2-D array (concatenate along first dimension)
  To Workspace9 : ToWorkspace  VariableName=RS  SaveFormat=Structure With Time  SampleTime=-1
      settings: Save2DSignal=2-D array (concatenate along first dimension)
  tag scope: PDERS1=global, PDERS2=global, PDERS3=global, PDERS4=global, QDERS1=global, QDERS2=global, QDERS3=global, QDERS4=global, VStar1=global, VStar2=global, VStar3=global, VStar4=global, dturb_level=global, thetaStar1=global, thetaStar2=global, thetaStar3=global, thetaStar4=global
  wires:
  Demux2/3 -> [PDERS3]  "PDER3*"
  Demux2/4 -> [PDERS4]  "PDER4*"
  Demux2/8 -> [QDERS4]  "QDER4*"
  Demux2/7 -> [QDERS3]  "QDER3*"
  Demux2/6 -> [QDERS2]  "QDER2*"
  Demux2/5 -> [QDERS1]  "QDER1*"
  Mux/1 -> "Data Processing, Identification and Control"/6, " Measurement Noise Added"/1(u)
  "Data Processing, Identification and Control"/2 -> [dturb_level]
  Demux2/1 -> [PDERS1]  "PDER1*"
  Demux2/2 -> [PDERS2]  "PDER2*"
  Demux3/2 -> Scope/2  "u2"
  Demux3/1 -> Scope/1  "u1"
  Demux3/5 -> Scope/5  "u5"
  Demux3/6 -> Scope/6  "u6"
  Demux3/7 -> Scope/7  "u7"
  Demux3/8 -> Scope/8  "u8"
  Demux3/4 -> Scope/4  "u4"
  Demux3/3 -> Scope/3  "u3"
  Simulation Time/1 -> "Data Processing, Identification and Control"/4
  [Pm] -> To Workspace3/1, Mux2/1, "Data Processing, Identification and Control"/2, Scope2/1
  "Data Processing, Identification and Control"/3 -> Demux1/1
  Demux1/2 -> [thetaStar2]  "theta2*"
  Demux1/1 -> [thetaStar1]  "theta1*"
  Demux1/5 -> [VStar1]  "V1*"
  Demux1/6 -> [VStar2]  "V2*"
  Demux1/7 -> [VStar3]  "V3*"
  Demux1/8 -> [VStar4]  "V4*"
  Demux1/4 -> [thetaStar4]  "theta4*"
  Demux1/3 -> [thetaStar3]  "theta3*"
  [freqs] -> To Workspace6/1, Delay6/1
  [msdata] -> To Workspace5/1, Delay5/1
  Delay1/1 -> Scope8/2, Demux2/1
  "Data Processing, Identification and Control"/4 -> Scope1/1  "Gain Margin"
  "Data Processing, Identification and Control"/5 -> Scope1/2  "Phase Margin"
  "Data Processing, Identification and Control"/6 -> Scope9/1, To Workspace9/1, Delay2/1
  Measurement Noise Level/1 -> " Measurement Noise Added"/2(nlevel)
  Delay2/1 -> Scope9/2, Scope4/1
  " Measurement Noise Added"/2(noise) -> [noise]
  " Measurement Noise Added"/1(y) -> Scope5/2, Delay7/1, "Data Processing, Identification and Control"/1
  Gain/1 -> To Workspace10/1, Demux3/1
  "Data Processing, Identification and Control"/7 -> Scope6/1, To Workspace2/1
  Demux4/2 -> Goto10/1  "PDER2*"
  Demux4/6 -> Goto15/1  "QDER4*"
  Demux4/3 -> Goto12/1  "PDER4*"
  Demux4/1 -> Goto18/1  "PDER1*"
  Demux4/5 -> Goto14/1  "QDER2*"
  Demux4/4 -> Goto13/1  "QDER1*"
  Delay3/1 -> Demux4/1
  "Data Processing, Identification and Control"/8 -> To Workspace1/1, Scope7/1, Delay4/1
  Mux1/1 -> Scope11/1
  "Data Processing, Identification and Control"/9 -> To Workspace/1, Scope10/1, Mux1/2  "One Step-Ahead Prediction Error"
  Delay4/1 -> Mux1/1  "Regression Error"
  "Data Processing, Identification and Control"/10 -> To Workspace7/1, Scope12/1
  Mux2/1 -> [PQ]
  From/1 -> Sum/1
  "Data Processing, Identification and Control"/1 -> Delay3/1, Scope8/1, Delay1/1, Sum/2
  Sum/1 -> Gain/1
  Delay5/1 -> Scope5/1, Mux/1
  Delay6/1 -> Mux/2
  Delay7/1 -> "Data Processing, Identification and Control"/5
  [Qm] -> To Workspace4/1, Mux2/2, Scope3/1, "Data Processing, Identification and Control"/3

== system MGTestSystem_4bus/Subsystem1 ==
  w : Inport
  V : Inport  Port=2
  w0 : Inport  Port=3
  V0 : Inport  Port=4
  Gain : Gain  Gain=Kp
  Gain1 : Gain  Gain=Kq
  Scope{1..4} (4 alike) : Scope  NumInputPorts=2
  Sum : Sum  Inputs=+++|
  Sum1 : Sum  Inputs=+-|
  Sum2 : Sum  Inputs=+++|
  Sum3 : Sum  Inputs=|-+
  Sum4 : Sum  Inputs=+-|
  Sum5 : Sum  Inputs=+-|
  Pref : Outport  VectorParamsAs1DForOutWhenUnconnected=off
  Qref : Outport  Port=2  VectorParamsAs1DForOutWhenUnconnected=off
  wires:
  [Qm4] -> Sum2/1, Sum5/2
  Sum2/1 -> Scope3/2, Qref/1
  Gain/1 -> Sum/2, Scope1/1
  Sum/1 -> Pref/1, Scope1/2
  Sum1/1 -> Gain/1, Scope4/2
  Gain1/1 -> Sum2/2, Scope3/1  "V*"
  Sum3/1 -> Gain1/1, Scope2/2
  w/1 -> Sum1/2, Scope4/1
  V/1 -> Sum3/1, Scope2/1
  V0/1 -> Sum3/2
  w0/1 -> Sum1/1
  [Pm4] -> Sum4/2, Sum/1
  [PDERS4] -> Sum4/1
  Sum4/1 -> Sum/3
  [QDERS4] -> Sum5/1
  Sum5/1 -> Sum2/3

== system MGTestSystem_4bus/Subsystem2 ==
  w : Inport
  V : Inport  Port=2
  w0 : Inport  Port=3
  V0 : Inport  Port=4
  Gain : Gain  Gain=Kp
  Gain1 : Gain  Gain=Kq
  Scope{1..4} (4 alike) : Scope  NumInputPorts=2
  Sum : Sum  Inputs=+++|
  Sum1 : Sum  Inputs=+-|
  Sum2 : Sum  Inputs=+++|
  Sum3 : Sum  Inputs=|-+
  Sum4 : Sum  Inputs=+-|
  Sum5 : Sum  Inputs=+-|
  Pref : Outport  VectorParamsAs1DForOutWhenUnconnected=off
  Qref : Outport  Port=2  VectorParamsAs1DForOutWhenUnconnected=off
  wires:
  [Qm2] -> Sum5/2, Sum2/1
  Sum2/1 -> Qref/1
  Gain/1 -> Sum/2, Scope1/1
  Sum/1 -> Pref/1, Scope1/2
  Sum1/1 -> Gain/1, Scope4/2
  Gain1/1 -> Sum2/2, Scope3/1  "V*"
  Sum3/1 -> Gain1/1, Scope2/2
  w/1 -> Sum1/2, Scope4/1
  V/1 -> Sum3/1, Scope2/1
  V0/1 -> Sum3/2
  w0/1 -> Sum1/1
  [Pm2] -> Sum4/2, Sum/1
  [PDERS2] -> Sum4/1
  Sum4/1 -> Sum/3
  [QDERS2] -> Sum5/1
  Sum5/1 -> Sum2/3

== system MGTestSystem_4bus/Bus_1/PLL ==
  Vabc_LN_pu : Inport
  2pi60'1 : Constant  Value=2*pi*60
  2pi60'2 : Constant  Value=2*pi*60
  2pi60'3 : Constant  Value=2*pi*60
  Constant : Constant  Value=90
  Demux : Demux  Outputs=3
  Gain1 : Gain  Gain=180/pi  SaturateOnIntegerOverflow=on  OutDataTypeStr=Inherit: Same as input  ParamDataTypeStr=Inherit: Same as input
  Gain2 : Gain  Gain=180/pi  SaturateOnIntegerOverflow=on  OutDataTypeStr=Inherit: Same as input  ParamDataTypeStr=Inherit: Same as input
  Gain3 : Gain  Gain=180/pi  SaturateOnIntegerOverflow=on  OutDataTypeStr=Inherit: Same as input  ParamDataTypeStr=Inherit: Same as input
  Mux : Mux  Inputs=3
  Pll1 : Subsystem
  Pll2 : Subsystem
  Pll3 : Subsystem
  Sum : Sum  Inputs=|++
  delta_abc : Outport  VectorParamsAs1DForOutWhenUnconnected=off
  wires:
  Vabc_LN_pu/1 -> Demux/1
  Demux/1 -> Pll3/1(señal)
  2pi60'3/1 -> Pll3/2(w)
  Pll3/1(f cos (rad)) -> Gain1/1
  Demux/2 -> Pll1/1(señal)
  2pi60'1/1 -> Pll1/2(w)
  Gain2/1 -> Mux/2
  Demux/3 -> Pll2/1(señal)
  2pi60'2/1 -> Pll2/2(w)
  Pll2/1(f cos (rad)) -> Gain3/1
  Gain3/1 -> Mux/3
  Pll1/1(f cos (rad)) -> Gain2/1
  Mux/1 -> Sum/1
  Gain1/1 -> Mux/1
  Constant/1 -> Sum/2
  Sum/1 -> delta_abc/1

== system MGTestSystem_4bus/Bus_1/Power Factor Block1 ==
  Vabc : Inport
  Iabc : Inport  Port=2
  Complex to Magnitude-Angle : ComplexToMagnitudeAngle
  Mux : Mux  Inputs=2
  Mux1 : Mux  Inputs=2
  Power : spsPowerLib/Power  Freq=Freq  Vinit=Vinit  Iinit=Iinit  Ts=Ts
      settings: SourceProductBaseCode=PS
  RMS3 : spsRMSLib/RMS  TrueRMS=on  Freq=60  RMSInit=0  Ts=Ts_Simulation
  RMS4 : spsRMSLib/RMS  TrueRMS=on  Freq=60  RMSInit=0  Ts=Ts_Simulation
  Real-Imag to Complex : RealImagToComplex
  Terminator : Terminator
  compara : Gain  SaturateOnIntegerOverflow=on  OutDataTypeStr=Inherit: Same as input  ParamDataTypeStr=Inherit: Same as input
  cos(theta) : Trigonometry  Operator=cos
  to Kw : Gain  Gain=1/1000
  to Kw1 : Gain  Gain=1/1000
  Pabc : Outport  VectorParamsAs1DForOutWhenUnconnected=off
  Qabc : Outport  Port=2  VectorParamsAs1DForOutWhenUnconnected=off
  Vabc y Vabc (rms) : Outport  Port=3  VectorParamsAs1DForOutWhenUnconnected=off
  Iabc y Iabc (rms) : Outport  Port=4  VectorParamsAs1DForOutWhenUnconnected=off
  "PFabc " : Outport  Port=5  VectorParamsAs1DForOutWhenUnconnected=off
  tag scope: P_abc_Bus2=global, Q_abc_Bus2=global
  wires:
  Complex to Magnitude-Angle/2 -> cos(theta)/1
  Real-Imag to Complex/1 -> Complex to Magnitude-Angle/1
  cos(theta)/1 -> "PFabc "/1
  Complex to Magnitude-Angle/1 -> Terminator/1
  Iabc/1 -> RMS4/1, compara/1, Power/2
  RMS4/1 -> Mux1/2
  Mux1/1 -> Iabc y Iabc (rms)/1
  Mux/1 -> Vabc y Vabc (rms)/1
  Vabc/1 -> Power/1, Mux/2, RMS3/1
  compara/1 -> Mux1/1
  RMS3/1 -> Mux/1
  Power/1 -> to Kw1/1, Pabc/1, Real-Imag to Complex/1
  Power/2 -> Qabc/1, Real-Imag to Complex/2, to Kw/1
  to Kw/1 -> [Q_abc_Bus2]
  to Kw1/1 -> [P_abc_Bus2]

== system MGTestSystem_4bus/Bus_2/PLL ==
  Vabc_LN_pu : Inport
  2pi60'1 : Constant  Value=2*pi*60
  2pi60'2 : Constant  Value=2*pi*60
  2pi60'3 : Constant  Value=2*pi*60
  Constant : Constant  Value=90
  Demux : Demux  Outputs=3
  Gain1 : Gain  Gain=180/pi  SaturateOnIntegerOverflow=on  OutDataTypeStr=Inherit: Same as input  ParamDataTypeStr=Inherit: Same as input
  Gain2 : Gain  Gain=180/pi  SaturateOnIntegerOverflow=on  OutDataTypeStr=Inherit: Same as input  ParamDataTypeStr=Inherit: Same as input
  Gain3 : Gain  Gain=180/pi  SaturateOnIntegerOverflow=on  OutDataTypeStr=Inherit: Same as input  ParamDataTypeStr=Inherit: Same as input
  Mux : Mux  Inputs=3
  Pll1 : Subsystem
  Pll2 : Subsystem
  Pll3 : Subsystem
  Sum : Sum  Inputs=|++
  delta_abc : Outport  VectorParamsAs1DForOutWhenUnconnected=off
  wires:
  Sum/1 -> delta_abc/1
  Constant/1 -> Sum/2
  Gain1/1 -> Mux/1
  Mux/1 -> Sum/1
  Pll1/1(f cos (rad)) -> Gain2/1
  Gain3/1 -> Mux/3
  Pll2/1(f cos (rad)) -> Gain3/1
  2pi60'2/1 -> Pll2/2(w)
  Demux/3 -> Pll2/1(señal)
  Gain2/1 -> Mux/2
  2pi60'1/1 -> Pll1/2(w)
  Demux/2 -> Pll1/1(señal)
  Pll3/1(f cos (rad)) -> Gain1/1
  2pi60'3/1 -> Pll3/2(w)
  Demux/1 -> Pll3/1(señal)
  Vabc_LN_pu/1 -> Demux/1

== system MGTestSystem_4bus/Bus_2/Power Factor Block1 ==
  Vabc : Inport
  Iabc : Inport  Port=2
  Complex to Magnitude-Angle : ComplexToMagnitudeAngle
  Mux : Mux  Inputs=2
  Mux1 : Mux  Inputs=2
  Power : spsPowerLib/Power  Freq=Freq  Vinit=Vinit  Iinit=Iinit  Ts=Ts
      settings: SourceProductBaseCode=PS
  RMS3 : spsRMSLib/RMS  TrueRMS=on  Freq=60  RMSInit=0  Ts=Ts_Simulation
  RMS4 : spsRMSLib/RMS  TrueRMS=on  Freq=60  RMSInit=0  Ts=Ts_Simulation
  Real-Imag to Complex : RealImagToComplex
  Terminator : Terminator
  compara : Gain  SaturateOnIntegerOverflow=on  OutDataTypeStr=Inherit: Same as input  ParamDataTypeStr=Inherit: Same as input
  cos(theta) : Trigonometry  Operator=cos
  to Kw : Gain  Gain=1/1000
  to Kw1 : Gain  Gain=1/1000
  Pabc : Outport  VectorParamsAs1DForOutWhenUnconnected=off
  Qabc : Outport  Port=2  VectorParamsAs1DForOutWhenUnconnected=off
  Vabc y Vabc (rms) : Outport  Port=3  VectorParamsAs1DForOutWhenUnconnected=off
  Iabc y Iabc (rms) : Outport  Port=4  VectorParamsAs1DForOutWhenUnconnected=off
  "PFabc " : Outport  Port=5  VectorParamsAs1DForOutWhenUnconnected=off
  tag scope: P_abc_Bus1=global, Q_abc_Bus1=global
  wires:
  to Kw1/1 -> [P_abc_Bus1]
  to Kw/1 -> [Q_abc_Bus1]
  Power/2 -> to Kw/1, Real-Imag to Complex/2, Qabc/1
  Power/1 -> Real-Imag to Complex/1, Pabc/1, to Kw1/1
  RMS3/1 -> Mux/1
  compara/1 -> Mux1/1
  Vabc/1 -> RMS3/1, Mux/2, Power/1
  Mux/1 -> Vabc y Vabc (rms)/1
  Mux1/1 -> Iabc y Iabc (rms)/1
  RMS4/1 -> Mux1/2
  Iabc/1 -> Power/2, compara/1, RMS4/1
  Complex to Magnitude-Angle/1 -> Terminator/1
  cos(theta)/1 -> "PFabc "/1
  Real-Imag to Complex/1 -> Complex to Magnitude-Angle/1
  Complex to Magnitude-Angle/2 -> cos(theta)/1

== system MGTestSystem_4bus/Bus_3/PLL ==
  Vabc_LN_pu : Inport
  2pi60'1 : Constant  Value=2*pi*60
  2pi60'2 : Constant  Value=2*pi*60
  2pi60'3 : Constant  Value=2*pi*60
  Constant : Constant  Value=90
  Demux : Demux  Outputs=3
  Gain1 : Gain  Gain=180/pi  SaturateOnIntegerOverflow=on  OutDataTypeStr=Inherit: Same as input  ParamDataTypeStr=Inherit: Same as input
  Gain2 : Gain  Gain=180/pi  SaturateOnIntegerOverflow=on  OutDataTypeStr=Inherit: Same as input  ParamDataTypeStr=Inherit: Same as input
  Gain3 : Gain  Gain=180/pi  SaturateOnIntegerOverflow=on  OutDataTypeStr=Inherit: Same as input  ParamDataTypeStr=Inherit: Same as input
  Mux : Mux  Inputs=3
  Pll1 : Subsystem
  Pll2 : Subsystem
  Pll3 : Subsystem
  Sum : Sum  Inputs=|++
  delta_abc : Outport  VectorParamsAs1DForOutWhenUnconnected=off
  wires:
  Sum/1 -> delta_abc/1
  Constant/1 -> Sum/2
  Gain1/1 -> Mux/1
  Mux/1 -> Sum/1
  Pll1/1(f cos (rad)) -> Gain2/1
  Gain3/1 -> Mux/3
  Pll2/1(f cos (rad)) -> Gain3/1
  2pi60'2/1 -> Pll2/2(w)
  Demux/3 -> Pll2/1(señal)
  Gain2/1 -> Mux/2
  2pi60'1/1 -> Pll1/2(w)
  Demux/2 -> Pll1/1(señal)
  Pll3/1(f cos (rad)) -> Gain1/1
  2pi60'3/1 -> Pll3/2(w)
  Demux/1 -> Pll3/1(señal)
  Vabc_LN_pu/1 -> Demux/1

== system MGTestSystem_4bus/Bus_3/Power Factor Block1 ==
  Vabc : Inport
  Iabc : Inport  Port=2
  Complex to Magnitude-Angle : ComplexToMagnitudeAngle
  Mux : Mux  Inputs=2
  Mux1 : Mux  Inputs=2
  Power : spsPowerLib/Power  Freq=Freq  Vinit=Vinit  Iinit=Iinit  Ts=Ts
      settings: SourceProductBaseCode=PS
  RMS3 : spsRMSLib/RMS  TrueRMS=on  Freq=60  RMSInit=0  Ts=Ts_Simulation
  RMS4 : spsRMSLib/RMS  TrueRMS=on  Freq=60  RMSInit=0  Ts=Ts_Simulation
  Real-Imag to Complex : RealImagToComplex
  Terminator : Terminator
  compara : Gain  SaturateOnIntegerOverflow=on  OutDataTypeStr=Inherit: Same as input  ParamDataTypeStr=Inherit: Same as input
  cos(theta) : Trigonometry  Operator=cos
  to Kw : Gain  Gain=1/1000
  to Kw1 : Gain  Gain=1/1000
  Pabc : Outport  VectorParamsAs1DForOutWhenUnconnected=off
  Qabc : Outport  Port=2  VectorParamsAs1DForOutWhenUnconnected=off
  Vabc y Vabc (rms) : Outport  Port=3  VectorParamsAs1DForOutWhenUnconnected=off
  Iabc y Iabc (rms) : Outport  Port=4  VectorParamsAs1DForOutWhenUnconnected=off
  "PFabc " : Outport  Port=5  VectorParamsAs1DForOutWhenUnconnected=off
  tag scope: P_abc_Bus3=global, Q_abc_Bus3=global
  wires:
  to Kw1/1 -> [P_abc_Bus3]
  to Kw/1 -> [Q_abc_Bus3]
  Power/2 -> to Kw/1, Real-Imag to Complex/2, Qabc/1
  Power/1 -> Real-Imag to Complex/1, Pabc/1, to Kw1/1
  RMS3/1 -> Mux/1
  compara/1 -> Mux1/1
  Vabc/1 -> RMS3/1, Mux/2, Power/1
  Mux/1 -> Vabc y Vabc (rms)/1
  Mux1/1 -> Iabc y Iabc (rms)/1
  RMS4/1 -> Mux1/2
  Iabc/1 -> Power/2, compara/1, RMS4/1
  Complex to Magnitude-Angle/1 -> Terminator/1
  cos(theta)/1 -> "PFabc "/1
  Real-Imag to Complex/1 -> Complex to Magnitude-Angle/1
  Complex to Magnitude-Angle/2 -> cos(theta)/1

== system MGTestSystem_4bus/Bus_4/PLL ==
  Vabc_LN_pu : Inport
  2pi60'1 : Constant  Value=2*pi*60
  2pi60'2 : Constant  Value=2*pi*60
  2pi60'3 : Constant  Value=2*pi*60
  Constant : Constant  Value=90
  Demux : Demux  Outputs=3
  Gain1 : Gain  Gain=180/pi  SaturateOnIntegerOverflow=on  OutDataTypeStr=Inherit: Same as input  ParamDataTypeStr=Inherit: Same as input
  Gain2 : Gain  Gain=180/pi  SaturateOnIntegerOverflow=on  OutDataTypeStr=Inherit: Same as input  ParamDataTypeStr=Inherit: Same as input
  Gain3 : Gain  Gain=180/pi  SaturateOnIntegerOverflow=on  OutDataTypeStr=Inherit: Same as input  ParamDataTypeStr=Inherit: Same as input
  Mux : Mux  Inputs=3
  Pll1 : Subsystem
  Pll2 : Subsystem
  Pll3 : Subsystem
  Sum : Sum  Inputs=|++
  delta_abc : Outport  VectorParamsAs1DForOutWhenUnconnected=off
  wires:
  Vabc_LN_pu/1 -> Demux/1
  Demux/1 -> Pll3/1(señal)
  2pi60'3/1 -> Pll3/2(w)
  Pll3/1(f cos (rad)) -> Gain1/1
  Demux/2 -> Pll1/1(señal)
  2pi60'1/1 -> Pll1/2(w)
  Gain2/1 -> Mux/2
  Demux/3 -> Pll2/1(señal)
  2pi60'2/1 -> Pll2/2(w)
  Pll2/1(f cos (rad)) -> Gain3/1
  Gain3/1 -> Mux/3
  Pll1/1(f cos (rad)) -> Gain2/1
  Mux/1 -> Sum/1
  Gain1/1 -> Mux/1
  Constant/1 -> Sum/2
  Sum/1 -> delta_abc/1

== system MGTestSystem_4bus/Bus_4/Power Factor Block1 ==
  Vabc : Inport
  Iabc : Inport  Port=2
  Complex to Magnitude-Angle : ComplexToMagnitudeAngle
  Mux : Mux  Inputs=2
  Mux1 : Mux  Inputs=2
  Power : spsPowerLib/Power  Freq=Freq  Vinit=Vinit  Iinit=Iinit  Ts=Ts
      settings: SourceProductBaseCode=PS
  RMS3 : spsRMSLib/RMS  TrueRMS=on  Freq=60  RMSInit=0  Ts=Ts_Simulation
  RMS4 : spsRMSLib/RMS  TrueRMS=on  Freq=60  RMSInit=0  Ts=Ts_Simulation
  Real-Imag to Complex : RealImagToComplex
  Terminator : Terminator
  compara : Gain  SaturateOnIntegerOverflow=on  OutDataTypeStr=Inherit: Same as input  ParamDataTypeStr=Inherit: Same as input
  cos(theta) : Trigonometry  Operator=cos
  to Kw : Gain  Gain=1/1000
  to Kw1 : Gain  Gain=1/1000
  Pabc : Outport  VectorParamsAs1DForOutWhenUnconnected=off
  Qabc : Outport  Port=2  VectorParamsAs1DForOutWhenUnconnected=off
  Vabc y Vabc (rms) : Outport  Port=3  VectorParamsAs1DForOutWhenUnconnected=off
  Iabc y Iabc (rms) : Outport  Port=4  VectorParamsAs1DForOutWhenUnconnected=off
  "PFabc " : Outport  Port=5  VectorParamsAs1DForOutWhenUnconnected=off
  tag scope: P_abc_Bus4=global, Q_abc_Bus4=global
  wires:
  Complex to Magnitude-Angle/2 -> cos(theta)/1
  Real-Imag to Complex/1 -> Complex to Magnitude-Angle/1
  cos(theta)/1 -> "PFabc "/1
  Complex to Magnitude-Angle/1 -> Terminator/1
  Iabc/1 -> RMS4/1, compara/1, Power/2
  RMS4/1 -> Mux1/2
  Mux1/1 -> Iabc y Iabc (rms)/1
  Mux/1 -> Vabc y Vabc (rms)/1
  Vabc/1 -> Power/1, Mux/2, RMS3/1
  compara/1 -> Mux1/1
  RMS3/1 -> Mux/1
  Power/1 -> to Kw1/1, Pabc/1, Real-Imag to Complex/1
  Power/2 -> Qabc/1, Real-Imag to Complex/2, to Kw/1
  to Kw/1 -> [Q_abc_Bus4]
  to Kw1/1 -> [P_abc_Bus4]
